simulink model "TestingGrounds"  (R2021a)
settings: Solver=VariableStepAuto  StartTime=0.0  StopTime=10.0  RelTol=1e-3
libraries: simulink x4, TrafficSimulationLibrary x1
settings Model: Creator=phill  LastModifiedBy=phill

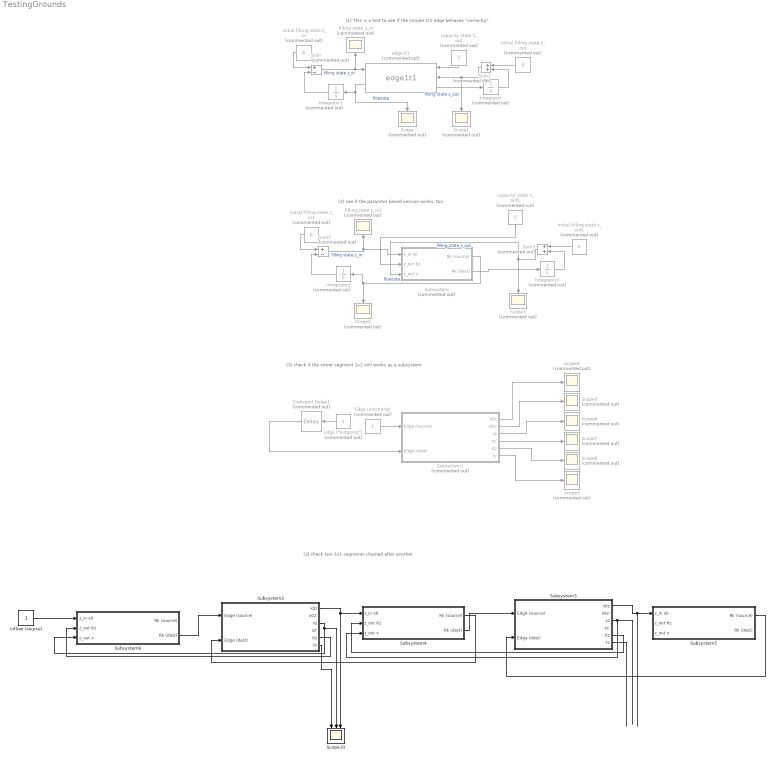
== system TestingGrounds ==
  note: (1) This is a test to see if the simple 1t1 edge behaves "correctly".
  note: (2) see if the paramter based version works, too
  note: (3) check if the street segment 1x1 still works as a subsystem
  note: (3) check two 1x1 segments chained after another
  "Edge (\"outgoing\")" : Constant  Commented=on
  Edge (incoming) : Constant  Commented=on
  Integrator{,1..3} (4 alike) : Integrator  Commented=on
  Scope{,1..9} (10 alike) : Scope  Commented=on
  Scope10 : Scope  NumInputPorts=3
  Subsystem : Subsystem  Commented=on  mask{Rk=1}
      mask prompts: Rk "Rk (fixed flowrate, used when the flow is enabled)"
      mask help: This block connects one source-cell [z_in] to one destination-cell [z_out], and prompts a flow of cars with the rate Rk (Parameter) if and only if there are still cars at the end of [z_out] avaiable and if the capacity of [z_out] is not yet surpassed, i.e. (z_in x0 > 0 AND z_out Kz > z_out x), otherwise the flow is reduced to 0.
      mask Display:
      | disp('Simple Edge 1x1 \n\n');
      | disp(['Rk = ', get_param(gcb,'Rk')])
  Subsystem1 : Subsystem  Commented=on  mask{Kz=10, Tz=3}
      mask prompts: Kz "Kz (Capacity - How many cars fit into this cell)"; Tz "Tz (Nominal travel time for vehicles traveling unobstructed through the cell)"
      mask help:
      | This Block models a single Street-Lane capable of holding / transducing cars (or at least "car volume units") as a cell. This 1x1 version It is connected to a single source edge (over which it can receive cars from a preceeding cell) and a single destination edge (over which it can lose cars to the succeeding cell).  It has a capacity (how many volume-units of cars can be present on the segment at a given time) and a nominal travel time (how long cars would need to travel through it unobstructed). The outputs are:
      |
      | x0z  : how many cars (in car volume units) are "at the end of the cell" (and thus visible for the destination-edge  or the following cell).  The value can only rise if more cars flow in (mind the delay Tz!) than flow out - for instance if a traffic light blocks the exit.
      | x0z' : how many cars flow into (when positive sign) or out of (when negative) the cell
      | xz    : how many cars are in the cell in total (both the ones who just entered and have not reached the end yet, as well as the ones at the end)
      | xz'   : how many cars are flowing into- (positive sign) or out of (negative) the cell per time
      | yz    : the internal flow - how many cars pass into the "endpart" of a cell. It is delayed by Tz compared to the incoming flow y_incoming, so any cars that enter a cell will only "appear visible" at the end of it after that time Tz.
      mask Display:
      | disp('Street Lane Segment 1x1 \n\n');
      | disp(['Kz = ', get_param(gcb,'Kz'), ' | Tz = ', get_param(gcb, 'Tz')])
  Subsystem2 : Subsystem  mask{Kz=5, Tz=3}
      mask prompts: Kz "Kz (Capacity - How many cars fit into this cell)"; Tz "Tz (Nominal travel time for vehicles traveling unobstructed through the cell)"
      mask help:
      | This Block models a single Street-Lane capable of holding / transducing cars (or at least "car volume units") as a cell. This 1x1 version It is connected to a single source edge (over which it can receive cars from a preceeding cell) and a single destination edge (over which it can lose cars to the succeeding cell).  It has a capacity (how many volume-units of cars can be present on the segment at a given time) and a nominal travel time (how long cars would need to travel through it unobstructed). The outputs are:
      |
      | x0z  : how many cars (in car volume units) are "at the end of the cell" (and thus visible for the destination-edge  or the following cell).  The value can only rise if more cars flow in (mind the delay Tz!) than flow out - for instance if a traffic light blocks the exit.
      | x0z' : how many cars flow into (when positive sign) or out of (when negative) the cell
      | xz    : how many cars are in the cell in total (both the ones who just entered and have not reached the end yet, as well as the ones at the end)
      | xz'   : how many cars are flowing into- (positive sign) or out of (negative) the cell per time
      | yz    : the internal flow - how many cars pass into the "endpart" of a cell. It is delayed by Tz compared to the incoming flow y_incoming, so any cars that enter a cell will only "appear visible" at the end of it after that time Tz.
      mask Display:
      | disp('Street Lane Segment 1x1 \n\n');
      | disp(['Kz = ', get_param(gcb,'Kz'), ' | Tz = ', get_param(gcb, 'Tz')])
  Subsystem3 : Subsystem  mask{Kz=5, Tz=3}
      mask prompts: Kz "Kz (Capacity - How many cars fit into this cell)"; Tz "Tz (Nominal travel time for vehicles traveling unobstructed through the cell)"
      mask help:
      | This Block models a single Street-Lane capable of holding / transducing cars (or at least "car volume units") as a cell. This 1x1 version It is connected to a single source edge (over which it can receive cars from a preceeding cell) and a single destination edge (over which it can lose cars to the succeeding cell).  It has a capacity (how many volume-units of cars can be present on the segment at a given time) and a nominal travel time (how long cars would need to travel through it unobstructed). The outputs are:
      |
      | x0z  : how many cars (in car volume units) are "at the end of the cell" (and thus visible for the destination-edge  or the following cell).  The value can only rise if more cars flow in (mind the delay Tz!) than flow out - for instance if a traffic light blocks the exit.
      | x0z' : how many cars flow into (when positive sign) or out of (when negative) the cell
      | xz    : how many cars are in the cell in total (both the ones who just entered and have not reached the end yet, as well as the ones at the end)
      | xz'   : how many cars are flowing into- (positive sign) or out of (negative) the cell per time
      | yz    : the internal flow - how many cars pass into the "endpart" of a cell. It is delayed by Tz compared to the incoming flow y_incoming, so any cars that enter a cell will only "appear visible" at the end of it after that time Tz.
      mask Display:
      | disp('Street Lane Segment 1x1 \n\n');
      | disp(['Kz = ', get_param(gcb,'Kz'), ' | Tz = ', get_param(gcb, 'Tz')])
  Subsystem4 : Subsystem  mask{Rk=1}
      mask prompts: Rk "Rk (fixed flowrate, used when the flow is enabled)"
      mask help: This block serves to establish a flow between two Street Lane Segments. To archieve this, it connects one source-cell [z_in] to one destination-cell [z_out], and prompts a flow of cars with the rate Rk (Parameter) if and only if there are still cars at the end of [z_out] avaiable and if the capacity of [z_out] is not yet surpassed, i.e. (z_in x0 > 0 AND z_out Kz > z_out x), otherwise the flow is reduced to 0.
      mask Display:
      | disp('Simple Edge 1x1 \n\n');
      | disp(['Rk = ', get_param(gcb,'Rk')])
  Subsystem5 : Subsystem  mask{Rk=1}
      mask prompts: Rk "Rk (fixed flowrate, used when the flow is enabled)"
      mask help: This block serves to establish a flow between two Street Lane Segments. To archieve this, it connects one source-cell [z_in] to one destination-cell [z_out], and prompts a flow of cars with the rate Rk (Parameter) if and only if there are still cars at the end of [z_out] avaiable and if the capacity of [z_out] is not yet surpassed, i.e. (z_in x0 > 0 AND z_out Kz > z_out x), otherwise the flow is reduced to 0.
      mask Display:
      | disp('Simple Edge 1x1 \n\n');
      | disp(['Rk = ', get_param(gcb,'Rk')])
  Subsystem6 : Subsystem  mask{Rk=1}
      mask prompts: Rk "Rk (fixed flowrate, used when the flow is enabled)"
      mask help: This block serves to establish a flow between two Street Lane Segments. To archieve this, it connects one source-cell [z_in] to one destination-cell [z_out], and prompts a flow of cars with the rate Rk (Parameter) if and only if there are still cars at the end of [z_out] avaiable and if the capacity of [z_out] is not yet surpassed, i.e. (z_in x0 > 0 AND z_out Kz > z_out x), otherwise the flow is reduced to 0.
      mask Display:
      | disp('Simple Edge 1x1 \n\n');
      | disp(['Rk = ', get_param(gcb,'Rk')])
  Sum : Sum  Commented=on  Inputs=+-
  Sum1 : Sum  Commented=on
  Sum2 : Sum  Commented=on  Inputs=+-
  Sum3 : Sum  Commented=on
  Transport Delay1 : TransportDelay  Commented=on  DelayTime=6
  capacity state z_out : Constant  Commented=on  Value=5
  capacity state z_out1 : Constant  Commented=on  Value=5
  edge1t1 : TrafficSimulationLibrary/edge1t1  Commented=on  SystemSampleTime=-1  VariantActivationTime=update diagram  Latency=0  AutoFrameSizeCalculation=off
      settings: PortSchema="{\"entries\":[{\"content\":{\"sides\":[{\"content\":{\"connectorIds\":[\"In1\",\"Out2\"]},\"type\":\"ConnectorPlacement.EquallySpacedRectSide\",\"uuid\":\"c437cf4c-79e4-403f-acc5-73d37113f26d\"},{\"content\":{\"connectorIds\":[\"In2\",\"In3\",\"Out1\"],\"side\":\"RIGHT\"},\"type\":\"ConnectorPlacement.EquallySpacedRectSide\",\"uuid\":\"b2176c48-3cc9-4030-bf6c-6d327e823efa\"},{\"content\":{\"connectorIds\":[],\"side\":\"TOP\"},\"type\":\"ConnectorPlacement.EquallySpacedRectSide\",\"uuid\":\"abeed986-5952-4b96-a6ed-dc33fbc723e6\"}]},\"type\":\"ConnectorPlacement.EquallySpacedConnector\",\"uuid\":\"f01997e7-23a3-4397-8121-8272fdaf74ca\"}],\"packageUris\":[\"http://schema.mathworks.com/mf0/Connector/R2020b\"],\"version\":\"1.0\"}"
  filling state z_in : Scope  Commented=on
  filling state z_in1 : Scope  Commented=on
  inflow (source) : Constant
  initial filling state z_in : Constant  Commented=on  Value=6
  initial filling state z_in1 : Constant  Commented=on  Value=6
  initial filling state z_out : Constant  Commented=on  Value=0
  initial filling state z_out1 : Constant  Commented=on  Value=0
  wires:
  Sum/1 -> edge1t1/1, filling state z_in/1  "filling state z_in"
  edge1t1/2 -> Integrator1/1, Scope/1  "flowrate"
  initial filling state z_in/1 -> Sum/1
  capacity state z_out/1 -> edge1t1/2
  Sum1/1 -> edge1t1/3, Scope1/1  "filling state z_out"
  initial filling state z_out/1 -> Sum1/1
  edge1t1/1 -> Integrator/1
  Integrator/1 -> Sum1/2
  Integrator1/1 -> Sum/2
  Subsystem/2(Rk (dest)) -> Integrator2/1
  Integrator3/1 -> Sum2/2
  capacity state z_out1/1 -> Subsystem/2(z_out Kz)
  Sum3/1 -> Scope3/1, Subsystem/3(z_out x)  "filling state z_out"
  Sum2/1 -> Subsystem/1(z_in x0), filling state z_in1/1  "filling state z_in"
  Integrator2/1 -> Sum3/2
  Subsystem/1(Rk (source)) -> Integrator3/1, Scope2/1  "flowrate"
  initial filling state z_out1/1 -> Sum3/1
  initial filling state z_in1/1 -> Sum2/1
  "Edge (\"outgoing\")"/1 -> Transport Delay1/1
  Transport Delay1/1 -> Subsystem1/2(Edge (dest))
  Edge (incoming)/1 -> Subsystem1/1(Edge (source))
  Subsystem1/1(x0z) -> Scope4/1
  Subsystem1/2(x0z') -> Scope5/1
  Subsystem1/3(xz) -> Scope6/1
  Subsystem1/4(xz') -> Scope7/1
  Subsystem1/5(Kz) -> Scope8/1
  Subsystem1/6(Yz) -> Scope9/1
  Subsystem6/2(Rk (dest)) -> Subsystem2/1(Edge (source))
  Subsystem4/1(Rk (source)) -> Subsystem2/2(Edge (dest))
  inflow (source)/1 -> Subsystem6/1(z_in x0)
  Subsystem2/5(Kz) -> Subsystem6/2(z_out Kz)
  Subsystem2/3(xz) -> Scope10/2, Subsystem6/3(z_out x)
  Subsystem2/1(x0z) -> Subsystem4/1(z_in x0), Scope10/3
  Subsystem3/5(Kz) -> Subsystem4/2(z_out Kz)
  Subsystem3/3(xz) -> Subsystem4/3(z_out x)
  Subsystem4/2(Rk (dest)) -> Subsystem3/1(Edge (source))
  Subsystem3/1(x0z) -> Subsystem5/1(z_in x0)
  Subsystem5/1(Rk (source)) -> Subsystem3/2(Edge (dest))
  Subsystem2/6(Yz) -> Scope10/1
  Subsystem3/6(Yz) -> ?

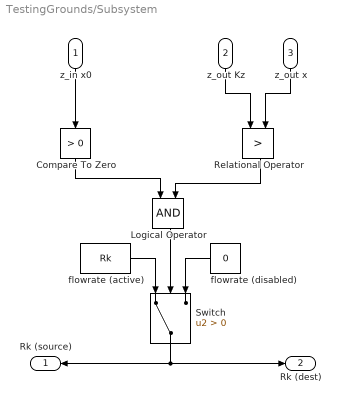
== system TestingGrounds/Subsystem ==
  z_in x0 : Inport
  z_out Kz : Inport  Port=2
  z_out x : Inport  Port=3
  Compare To Zero : simulink/Logic and Bit Operations/Compare To Zero  relop=>  OutDataTypeStr=boolean
  Logical Operator : Logic  AllPortsSameDT=off  OutDataTypeStr=boolean
  Relational Operator : RelationalOperator  Operator=>  OutDataTypeStr=boolean  RndMeth=Simplest
  Switch : Switch  Criteria=u2 > Threshold
  flowrate (active) : Constant  Value=Rk
  flowrate (disabled) : Constant  Value=0
  Rk (source) : Outport
  Rk (dest) : Outport  Port=2
  wires:
  flowrate (disabled)/1 -> Switch/3
  z_in x0/1 -> Compare To Zero/1
  Relational Operator/1 -> Logical Operator/2
  flowrate (active)/1 -> Switch/1
  Switch/1 -> Rk (dest)/1, Rk (source)/1
  z_out Kz/1 -> Relational Operator/1
  Logical Operator/1 -> Switch/2
  z_out x/1 -> Relational Operator/2
  Compare To Zero/1 -> Logical Operator/1

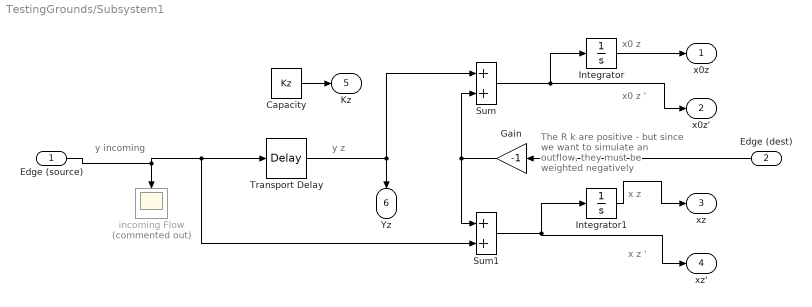
== system TestingGrounds/Subsystem1 ==
  note: y incoming
  note: x z '
  note: x z
  note: x0 z
  note: x0 z '
  note: y z
  note: The R k are positive - but since we
      | want to simulate an outflow, they
      | must be weighted negatively
  Edge (source) : Inport
  Edge (dest) : Inport  Port=2
  Capacity : Constant  Value=Kz
  Gain : Gain  Gain=-1
  Integrator : Integrator
  Integrator1 : Integrator
  Sum : Sum
  Sum1 : Sum
  Transport Delay : TransportDelay  DelayTime=Tz
  incoming Flow : Scope  Commented=on
  x0z : Outport
  x0z' : Outport  Port=2
  xz : Outport  Port=3
  xz' : Outport  Port=4
  Kz : Outport  Port=5
  Yz : Outport  Port=6
  wires:
  Sum1/1 -> xz'/1, Integrator1/1
  Integrator/1 -> x0z/1
  Transport Delay/1 -> Yz/1, Sum/1
  Edge (dest)/1 -> Gain/1
  Edge (source)/1 -> Sum1/2, Transport Delay/1, incoming Flow/1
  Integrator1/1 -> xz/1
  Gain/1 -> Sum1/1, Sum/2
  Sum/1 -> x0z'/1, Integrator/1
  Capacity/1 -> Kz/1

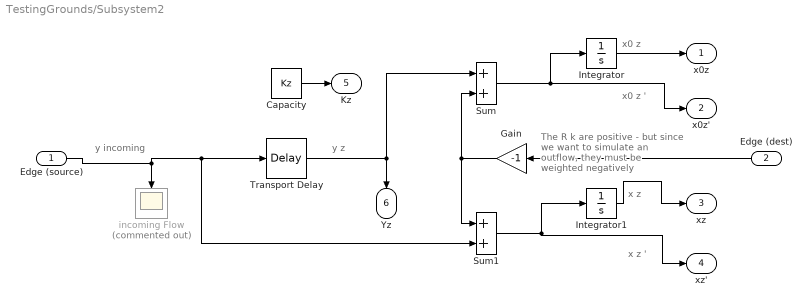
== system TestingGrounds/Subsystem2 ==
  note: y incoming
  note: x z '
  note: x z
  note: x0 z
  note: x0 z '
  note: y z
  note: The R k are positive - but since we
      | want to simulate an outflow, they
      | must be weighted negatively
  Edge (source) : Inport
  Edge (dest) : Inport  Port=2
  Capacity : Constant  Value=Kz
  Gain : Gain  Gain=-1
  Integrator : Integrator
  Integrator1 : Integrator
  Sum : Sum
  Sum1 : Sum
  Transport Delay : TransportDelay  DelayTime=Tz
  incoming Flow : Scope  Commented=on
  x0z : Outport
  x0z' : Outport  Port=2
  xz : Outport  Port=3
  xz' : Outport  Port=4
  Kz : Outport  Port=5
  Yz : Outport  Port=6
  wires:
  Sum1/1 -> xz'/1, Integrator1/1
  Integrator/1 -> x0z/1
  Transport Delay/1 -> Yz/1, Sum/1
  Edge (dest)/1 -> Gain/1
  Edge (source)/1 -> Sum1/2, Transport Delay/1, incoming Flow/1
  Integrator1/1 -> xz/1
  Gain/1 -> Sum1/1, Sum/2
  Sum/1 -> x0z'/1, Integrator/1
  Capacity/1 -> Kz/1

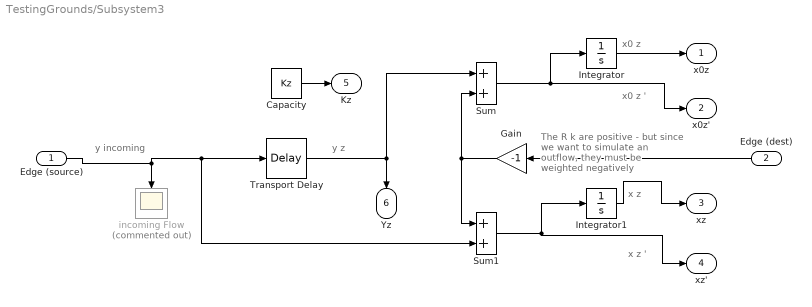
== system TestingGrounds/Subsystem3 ==
  note: y incoming
  note: x z '
  note: x z
  note: x0 z
  note: x0 z '
  note: y z
  note: The R k are positive - but since we
      | want to simulate an outflow, they
      | must be weighted negatively
  Edge (source) : Inport
  Edge (dest) : Inport  Port=2
  Capacity : Constant  Value=Kz
  Gain : Gain  Gain=-1
  Integrator : Integrator
  Integrator1 : Integrator
  Sum : Sum
  Sum1 : Sum
  Transport Delay : TransportDelay  DelayTime=Tz
  incoming Flow : Scope  Commented=on
  x0z : Outport
  x0z' : Outport  Port=2
  xz : Outport  Port=3
  xz' : Outport  Port=4
  Kz : Outport  Port=5
  Yz : Outport  Port=6
  wires:
  Sum1/1 -> xz'/1, Integrator1/1
  Integrator/1 -> x0z/1
  Transport Delay/1 -> Yz/1, Sum/1
  Edge (dest)/1 -> Gain/1
  Edge (source)/1 -> Sum1/2, Transport Delay/1, incoming Flow/1
  Integrator1/1 -> xz/1
  Gain/1 -> Sum1/1, Sum/2
  Sum/1 -> x0z'/1, Integrator/1
  Capacity/1 -> Kz/1

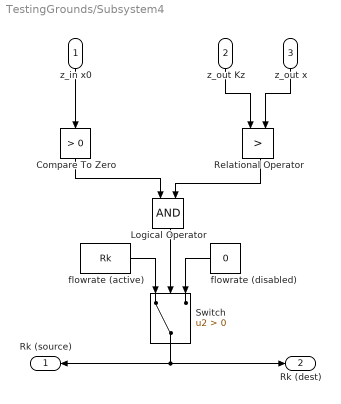
== system TestingGrounds/Subsystem4 ==
  z_in x0 : Inport
  z_out Kz : Inport  Port=2
  z_out x : Inport  Port=3
  Compare To Zero : simulink/Logic and Bit Operations/Compare To Zero  relop=>  OutDataTypeStr=boolean
  Logical Operator : Logic  AllPortsSameDT=off  OutDataTypeStr=boolean
  Relational Operator : RelationalOperator  Operator=>  OutDataTypeStr=boolean  RndMeth=Simplest
  Switch : Switch  Criteria=u2 > Threshold
  flowrate (active) : Constant  Value=Rk
  flowrate (disabled) : Constant  Value=0
  Rk (source) : Outport
  Rk (dest) : Outport  Port=2
  wires:
  flowrate (disabled)/1 -> Switch/3
  z_in x0/1 -> Compare To Zero/1
  Relational Operator/1 -> Logical Operator/2
  flowrate (active)/1 -> Switch/1
  Switch/1 -> Rk (dest)/1, Rk (source)/1
  z_out Kz/1 -> Relational Operator/1
  Logical Operator/1 -> Switch/2
  z_out x/1 -> Relational Operator/2
  Compare To Zero/1 -> Logical Operator/1

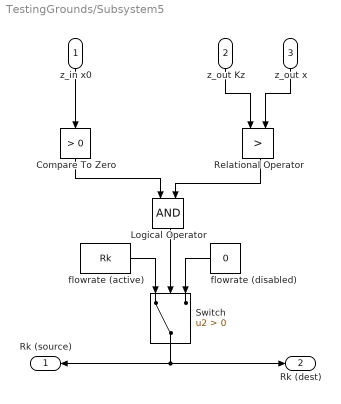
== system TestingGrounds/Subsystem5 ==
  z_in x0 : Inport
  z_out Kz : Inport  Port=2
  z_out x : Inport  Port=3
  Compare To Zero : simulink/Logic and Bit Operations/Compare To Zero  relop=>  OutDataTypeStr=boolean
  Logical Operator : Logic  AllPortsSameDT=off  OutDataTypeStr=boolean
  Relational Operator : RelationalOperator  Operator=>  OutDataTypeStr=boolean  RndMeth=Simplest
  Switch : Switch  Criteria=u2 > Threshold
  flowrate (active) : Constant  Value=Rk
  flowrate (disabled) : Constant  Value=0
  Rk (source) : Outport
  Rk (dest) : Outport  Port=2
  wires:
  flowrate (disabled)/1 -> Switch/3
  z_in x0/1 -> Compare To Zero/1
  Relational Operator/1 -> Logical Operator/2
  flowrate (active)/1 -> Switch/1
  Switch/1 -> Rk (dest)/1, Rk (source)/1
  z_out Kz/1 -> Relational Operator/1
  Logical Operator/1 -> Switch/2
  z_out x/1 -> Relational Operator/2
  Compare To Zero/1 -> Logical Operator/1

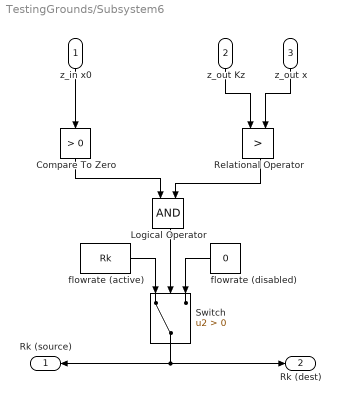
== system TestingGrounds/Subsystem6 ==
  z_in x0 : Inport
  z_out Kz : Inport  Port=2
  z_out x : Inport  Port=3
  Compare To Zero : simulink/Logic and Bit Operations/Compare To Zero  relop=>  OutDataTypeStr=boolean
  Logical Operator : Logic  AllPortsSameDT=off  OutDataTypeStr=boolean
  Relational Operator : RelationalOperator  Operator=>  OutDataTypeStr=boolean  RndMeth=Simplest
  Switch : Switch  Criteria=u2 > Threshold
  flowrate (active) : Constant  Value=Rk
  flowrate (disabled) : Constant  Value=0
  Rk (source) : Outport
  Rk (dest) : Outport  Port=2
  wires:
  flowrate (disabled)/1 -> Switch/3
  z_in x0/1 -> Compare To Zero/1
  Relational Operator/1 -> Logical Operator/2
  flowrate (active)/1 -> Switch/1
  Switch/1 -> Rk (dest)/1, Rk (source)/1
  z_out Kz/1 -> Relational Operator/1
  Logical Operator/1 -> Switch/2
  z_out x/1 -> Relational Operator/2
  Compare To Zero/1 -> Logical Operator/1
